simulink model "Beautiful_powertrain"  (R2024a)
settings: Solver=ode3  StartTime=0.0  StopTime=40  FixedStep=0.001  RelTol=1e-3
model workspace (MAT data in the model file):
  C_Aero_drag = 0.28
  C_rolling_resistance = 0.01
  C_rolling_resitance = 0.01
  C_viscous_damping = 0.02
  Damping_coef = 50
  Gear_ratio = 10
  J_vehicle = 2.56328
  Motor_no_load_speed = 16000
  Motor_rated_load = 150000
  Motor_rated_speed = 9000
  Motor_rotor_damping = 0.02
  Motor_rotor_inertia = 0.05
  Motor_voltage = 450
  Slope = 0
  Vehicle_Wheel_Radius = 0.358
  Vehicle_frontal_area = 2.56
  Vehicle_mass = 2000
values from neighbouring files (symbols this model uses):
  s = sprintf('    [N_diangostic_2.m]
undefined symbols (not defined in the file or in its folder): battery_builder_rtmsupport, gcbh
libraries: Batteries_lib x36, fl_lib x31, nesl_utility x24, ee_lib x3, autolibshared x2, rllib x2, sdl_lib x1
(part 1 of 6)
settings Model: Creator=bt  LastModifiedBy=konstantinosspiliotopoulos
settings SolverCC: AutoInsertRateTranBlk=on

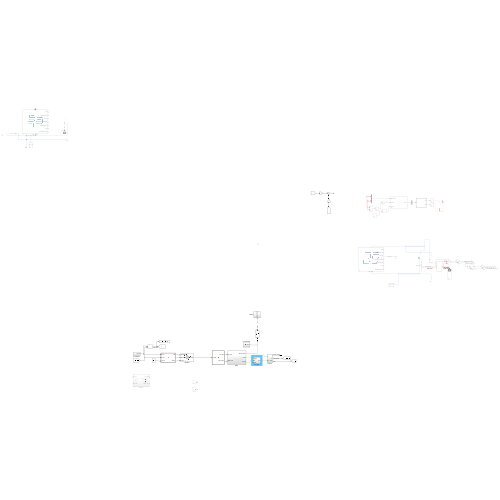
[thumbnail: Simulink's stored preview of the top-level diagram]
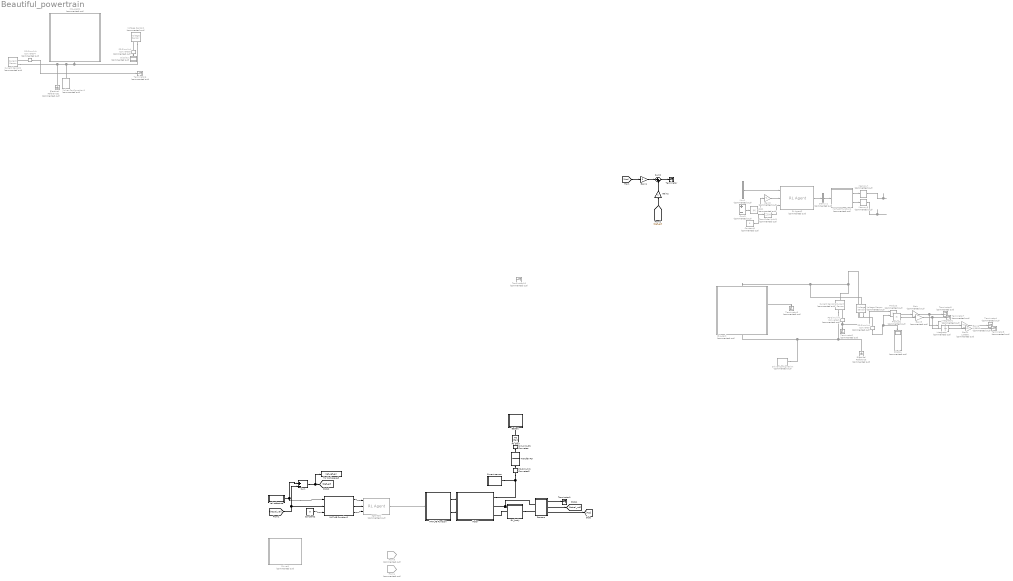
== system Beautiful_powertrain ==
  Abs1 : Abs  Commented=on  SaturateOnIntegerOverflow=off
  Battery : Subsystem
  Constant1 : Constant  Commented=on  Value=0
  Constant2 : Constant  Value=0
  Current Sensor : fl_lib/Electrical/Electrical Sensors/Current Sensor  Commented=on
  Current Sensor2 : fl_lib/Electrical/Electrical Sensors/Current Sensor  Commented=on
  Current sensor : Subsystem
  Demux1 : Demux  Commented=on  Outputs=1
  Display : Display  Commented=on
  Display1 : Display  Commented=on
  Driver1 : Subsystem  Commented=on
  EV_body : Subsystem
  Electrical Reference : fl_lib/Electrical/Electrical Elements/Electrical Reference  Commented=on
  Electrical Reference1 : fl_lib/Electrical/Electrical Elements/Electrical Reference  Commented=on
  From3 : From  Commented=on  GotoTag=Vel_ref
  From4 : From  Commented=on  GotoTag=vel_act
  Gain : Gain  Commented=on  Gain=1e-3
  Gain1 : Gain
  Gain2 : Gain
  Gain3 : Gain  Commented=on  Gain=-1
  Gain4 : Gain  Commented=on  Gain=1/3600
  Gain5 : Gain  Commented=on  Gain=1e-3
  Gain6 : Gain  Commented=on  Gain=1/3600
  ID4_pack : Subsystem  Commented=on  LoadFcn=battery_builder_rtmsupport('loadfcn',gcbh);
      settings: CopyFcn=battery_builder_rtmsupport('copyfcn',gcbh);  PreCopyFcn=battery_builder_rtmsupport('precopyfcn',gcbh);  PreDeleteFcn=battery_builder_rtmsupport('predeletefcn',gcbh);  PortSchema="{\"entries\":[{\"content\":{\"sides\":[{\"content\":{\"connectorIds\":[\"LConn1\"]},\"type\":\"ConnectorPlacement.EquallySpacedRectSide\",\"uuid\":\"ff832d46-24c2-48f3-9ca2-acbc79ffea0e\"},{\"content\":{\"connectorIds\":[\"RConn1\"],\"side\":\"RIGHT\"},\"type\":\"ConnectorPlacement.EquallySpacedRectSide\",\"uuid\":\"f1f3b13c-36d9-4e7c-bb66-ad6aba201785\"},{\"content\":{\"side\":\"TOP\"},\"type\":\"ConnectorPlacement.EquallySpacedRectSide\",\"uuid\":\"497ed55c-0d21-4aaa-b04e-04d199c99403\"},{\"content\":{\"connectorIds\":[\"Out1\",\"Out2\",\"Out3\",\"Out4\",\"Out5\",\"Out6\",\"Out7\"],\"side\":\"BOTTOM\"},\"type\":\"ConnectorPlacement.EquallySpacedRectSide\",\"uuid\":\"fb4a2477-79f0-4aed-96ce-fa2286ad26a5\"}]},\"type\":\"ConnectorPlacement.EquallySpacedConnector\",\"uuid\":\"b44e404e-c709-4efd-83da-0fbfd4cccfd0\"}],\"packageUris\":[\"http://schema.mathworks.com/mf0/Connector/R2020b\"],\"version\":\"1.0\"}"
      mask Display: image('$imagefile')
  ID4_pack1 : Subsystem  Commented=on  LoadFcn=battery_builder_rtmsupport('loadfcn',gcbh);
      settings: CopyFcn=battery_builder_rtmsupport('copyfcn',gcbh);  PreCopyFcn=battery_builder_rtmsupport('precopyfcn',gcbh);  PreDeleteFcn=battery_builder_rtmsupport('predeletefcn',gcbh);  PortSchema="{\"entries\":[{\"content\":{\"sides\":[{\"content\":{\"connectorIds\":[\"LConn1\"]},\"type\":\"ConnectorPlacement.EquallySpacedRectSide\",\"uuid\":\"ff832d46-24c2-48f3-9ca2-acbc79ffea0e\"},{\"content\":{\"connectorIds\":[\"RConn1\"],\"side\":\"RIGHT\"},\"type\":\"ConnectorPlacement.EquallySpacedRectSide\",\"uuid\":\"f1f3b13c-36d9-4e7c-bb66-ad6aba201785\"},{\"content\":{\"side\":\"TOP\"},\"type\":\"ConnectorPlacement.EquallySpacedRectSide\",\"uuid\":\"497ed55c-0d21-4aaa-b04e-04d199c99403\"},{\"content\":{\"connectorIds\":[\"Out1\",\"Out2\",\"Out3\",\"Out4\",\"Out5\",\"Out6\",\"Out7\"],\"side\":\"BOTTOM\"},\"type\":\"ConnectorPlacement.EquallySpacedRectSide\",\"uuid\":\"fb4a2477-79f0-4aed-96ce-fa2286ad26a5\"}]},\"type\":\"ConnectorPlacement.EquallySpacedConnector\",\"uuid\":\"b44e404e-c709-4efd-83da-0fbfd4cccfd0\"}],\"packageUris\":[\"http://schema.mathworks.com/mf0/Connector/R2020b\"],\"version\":\"1.0\"}"
      mask Display: image('$imagefile')
  Integrator : Integrator  Commented=on
  Integrator1 : Integrator  Commented=on
  MATLAB Function : MATLAB Function  TreatAsAtomicUnit=on
  MATLAB Function1 : MATLAB Function  Commented=on  TreatAsAtomicUnit=on
  MATLAB Function2 : MATLAB Function  TreatAsAtomicUnit=on
  Memory2 : Memory  Commented=on
  Memory3 : Memory  Commented=on
  Motor : Subsystem
  Mux1 : Mux  Commented=on  Inputs=2
  PS Gain : fl_lib/Physical Signals/Functions/PS Gain  gain=1
  PS-Simulink Converter{,1,3..4} (4 alike) : nesl_utility/PS-Simulink Converter  Commented=on  PhysicalDomain=network_engine_domain  SubClassName=ps_output  LeftPortType=input  RightPortType=output  PseudoPeriodic=off  Frequencies=[]  VectorFormat=inherit  Unit=inherit  AffineConversion=off
  PS-Simulink Converter2 : nesl_utility/PS-Simulink Converter  PhysicalDomain=network_engine_domain  SubClassName=ps_output  LeftPortType=input  RightPortType=output  PseudoPeriodic=off  Frequencies=[]  VectorFormat=inherit  Unit=inherit  AffineConversion=off
  Product : Product  Commented=on
  Product1 : Product  Commented=on
  RL Agent2 : rllib/RL Agent  Commented=on  Agent=agentObj  ExternalActionAsInput=off  ProvideLastAction=off  ProvideCumRwd=off  TreatAsDirectFeedthrough=on  UseStrictObservationDataTypes=off
  Sensors : Subsystem
  Simulink-PS Converter : nesl_utility/Simulink-PS Converter  PhysicalDomain=network_engine_domain  SubClassName=ps_input  LeftPortType=input  RightPortType=output  PseudoPeriodic=off  Frequencies=[]  NoiseDistribution=none  NoiseParameters=[]  Unit=1  AffineConversion=off  FilteringAndDerivatives=provide  SimscapeFilterOrder=1  InputFilterTimeConstant=0.001  UdotUserProvided=0
  Solver Configuration : nesl_utility/Solver Configuration  Commented=on  PhysicalDomain=network_engine_domain  SubClassName=solver  LeftPortType=input  RightPortType=generic  Tones=[]  Harmonics=[]  SimulateNoise=off  Profile=off  UseLocalSampling=off  EnableSwitchedLinearOptims=on  FrequencyDomain=off  UseCCode=off  RelTol=0.001  AbsTol=0.001  MinStep=1e-09  ToWorkspace=off  RevertToSquareIcSolve=off  NumHomotopyIterations=100  PhasorMode=off  PhasorModeNumHarmonics=1  ConsistencySolver=NEWTON_XTOL_AFTER_FTOL  IndexReductionMethod=DerivativeReplacement  DoDC=off  ResidualTolerance=1e-09  ConsistencyTolSource=GLOBAL  ConsistencyAbsTol=0.001  ConsistencyRelTol=0.001  ConsistencyTolFactor=0.001  UseLocalSolver=off  LocalSolverChoice=NE_BACKWARD_EULER_ADVANCER  ResolveIndetEquations=on  FunctionEvalNumThread=1  LocalSolverSampleTime=0.001  DoFixedCost=off  MaxNonlinIter=3  MaxModeIter=2  ComputeImpulses=off  ImpulseIterations=2  LinearAlgebra=auto  LinearAlgebraNumThread=0  EquationFormulation=NE_TIME_EF  DelaysMemoryBudget=1024  AutomaticFiltering=on  FilteringTimeConstant=0.001  PartitionStorageMethod=AS_NEEDED  PartitionMemoryBudget=1024  PartitionMethod=ROBUST  MultibodyUseLocalSolver=off  MultibodyLocalSolverChoice=ODE1  MultibodyLocalSolverSampleTime=0.001
  Solver Configuration1 : nesl_utility/Solver Configuration  Commented=on  PhysicalDomain=network_engine_domain  SubClassName=solver  LeftPortType=input  RightPortType=generic  Tones=[]  Harmonics=[]  SimulateNoise=off  Profile=off  UseLocalSampling=off  EnableSwitchedLinearOptims=on  FrequencyDomain=off  UseCCode=off  RelTol=0.001  AbsTol=0.001  MinStep=1e-09  ToWorkspace=off  RevertToSquareIcSolve=off  NumHomotopyIterations=100  PhasorMode=off  PhasorModeNumHarmonics=1  ConsistencySolver=NEWTON_XTOL_AFTER_FTOL  IndexReductionMethod=DerivativeReplacement  DoDC=off  ResidualTolerance=1e-09  ConsistencyTolSource=GLOBAL  ConsistencyAbsTol=0.001  ConsistencyRelTol=0.001  ConsistencyTolFactor=0.001  UseLocalSolver=off  LocalSolverChoice=NE_BACKWARD_EULER_ADVANCER  ResolveIndetEquations=on  FunctionEvalNumThread=1  LocalSolverSampleTime=0.001  DoFixedCost=off  MaxNonlinIter=3  MaxModeIter=2  ComputeImpulses=off  ImpulseIterations=2  LinearAlgebra=auto  LinearAlgebraNumThread=0  EquationFormulation=NE_TIME_EF  DelaysMemoryBudget=1024  AutomaticFiltering=on  FilteringTimeConstant=0.001  PartitionStorageMethod=AS_NEEDED  PartitionMemoryBudget=1024  PartitionMethod=ROBUST  MultibodyUseLocalSolver=off  MultibodyLocalSolverChoice=ODE1  MultibodyLocalSolverSampleTime=0.001
  Sum : Sum  Inputs=|+-
  Sum2 : Sum  Inputs=|++
  Sum3 : Sum  Commented=on  Inputs=+-
  Terminator : Terminator
  Terminator1 : Terminator
  Terminator{2..8,10} (8 alike) : Terminator  Commented=on
  To Workspace3 : ToWorkspace  VariableName=Veh_ref_err  SaveFormat=Structure With Time  SampleTime=-1
  Transfer Fcn : TransferFcn  Denominator=[1e-2 1]
  Vel reference : Subsystem
  Voltage Sensor : fl_lib/Electrical/Electrical Sensors/Voltage Sensor  Commented=on
  Voltage Sensor1 : fl_lib/Electrical/Electrical Sensors/Voltage Sensor  Commented=on
  Zero-Order Hold1 : ZeroOrderHold  Commented=on  SampleTime=-1
  agentObj : rllib/RL Agent  Commented=on  Agent=agentObj  ExternalActionAsInput=off  ProvideLastAction=off  ProvideCumRwd=off  TreatAsDirectFeedthrough=on  UseStrictObservationDataTypes=off
  wires:
  Sensors/3(ACC) -> [Acc]  "ACC"
  [Acc] -> Gain1/1
  Gain1/1 -> Sum2/1
  Gain2/1 -> Sum2/2
  Sum2/1 -> Terminator/1
  Vel reference/1(Vel_ref) -> MATLAB Function2/1(Vel_ref), Sum/1
  [Actual_vel] -> Sum/2, MATLAB Function2/2(Vel_act)
  Memory3/1 -> ?
  MATLAB Function1/2(brk) -> Memory3/1
  Memory2/1 -> ?
  MATLAB Function1/1(acc) -> Memory2/1
  Demux1/1 -> MATLAB Function1/1(u)
  RL Agent2/1 -> Demux1/1
  Zero-Order Hold1/1 -> RL Agent2/3
  Constant1/1 -> Zero-Order Hold1/1
  Gain3/1 -> RL Agent2/2
  Abs1/1 -> Gain3/1
  Sum3/1 -> Abs1/1
  Mux1/1 -> RL Agent2/1
  ? -> Sum3/2
  ? -> Mux1/2
  ? -> Sum3/1
  ? -> Mux1/1
  Sensors/1(I) -> Terminator1/1  "Motor_omega"
  Sensors/2(O) -> [Actual_vel]  "ACTUAL VEL"
  Sum/1 -> To Workspace3/1, [Ref_err]  "REF_ERR"
  [Ref_err] -> Gain2/1
  PS-Simulink Converter/1 -> Product/2, Display/1  "Bat_Voltage"
  PS-Simulink Converter1/1 -> Terminator2/1, Product/1  "Bat_current"
  Product/1 -> Gain/1
  Gain/1 -> Integrator/1, Terminator3/1  "Bat_power [kW]"
  Integrator/1 -> Gain4/1
  Gain4/1 -> Terminator4/1  "Energy used [kWh]"
  PS-Simulink Converter2/1 -> Transfer Fcn/1
  Transfer Fcn/1 -> Simulink-PS Converter/1
  ID4_pack/3(socCell) -> Terminator5/1  "Bat_soc"
  PS-Simulink Converter3/1 -> Display1/1  "Bat_V"
  PS-Simulink Converter4/1 -> Terminator6/1  "Bat_I"
  ? -> Product1/2  "Bat_Voltage"
  Gain5/1 -> Integrator1/1, Terminator7/1  "Bat_power [kW]"
  ? -> ?  "Bat_Voltage"
  Product1/1 -> Gain5/1
  ? -> Product1/1  "Bat_current"
  Gain6/1 -> Terminator8/1  "Energy used [kWh]"
  Integrator1/1 -> Gain6/1
  MATLAB Function/1(Acc_cmd) -> Motor/1(Acc_cmd)
  MATLAB Function/2(Brake_cmd) -> Motor/2(Brake_cmd)
  Constant2/1 -> MATLAB Function2/3(u_used)
  MATLAB Function2/1(obs) -> agentObj/1
  MATLAB Function2/2(r) -> agentObj/2
  MATLAB Function2/3(isdone) -> agentObj/3
  agentObj/1 -> MATLAB Function/1(u_scalar)
  connections:
  Motor/RConn1 -- Current sensor/LConn1 -- PS-Simulink Converter2/LConn1
  EV_body/LConn1 -- Sensors/LConn1 -- Motor/RConn2
  EV_body/LConn2 -- Motor/RConn3
  EV_body/RConn1 -- Sensors/LConn2
  Electrical Reference/LConn1 -- Current Sensor/RConn2 -- Solver Configuration/RConn1 -- ID4_pack/RConn1
  PS-Simulink Converter/LConn1 -- Voltage Sensor/RConn1
  Voltage Sensor/LConn1 -- ID4_pack/LConn1 -- Current Sensor/LConn1 -- Voltage Sensor/RConn2
  PS-Simulink Converter1/LConn1 -- Current Sensor/RConn1
  Simulink-PS Converter/RConn1 -- PS Gain/LConn1
  Electrical Reference1/LConn1 -- Current Sensor2/RConn2 -- Voltage Sensor1/RConn2 -- ID4_pack1/RConn1 -- Solver Configuration1/RConn1
  PS-Simulink Converter3/LConn1 -- Voltage Sensor1/RConn1
  PS-Simulink Converter4/LConn1 -- Current Sensor2/RConn1
  PS Gain/RConn1 -- Battery/RConn1

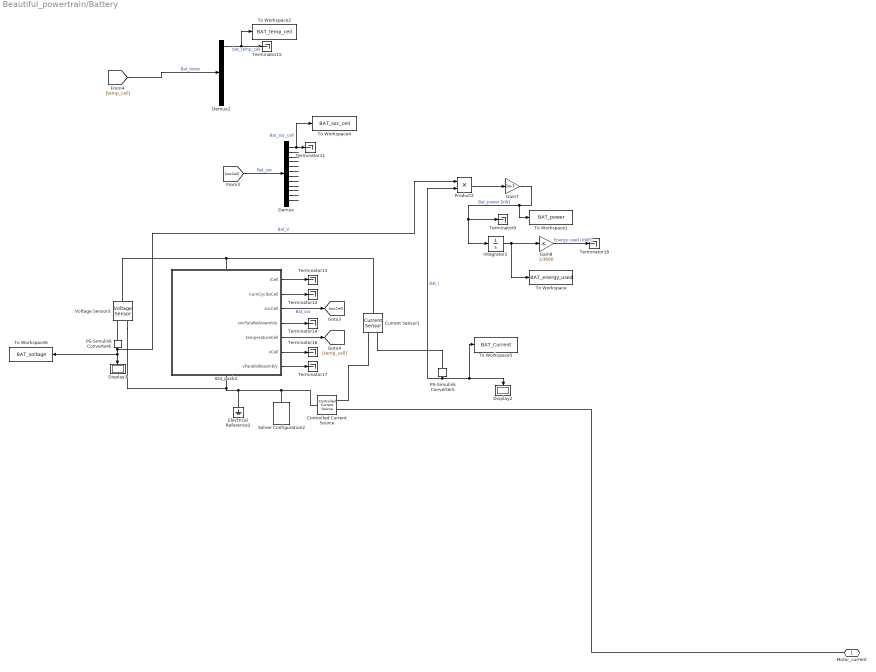
== system Beautiful_powertrain/Battery ==
  Controlled Current Source : fl_lib/Electrical/Electrical Sources/Controlled Current Source
  Current Sensor1 : fl_lib/Electrical/Electrical Sensors/Current Sensor
  Demux : Demux  Outputs=12
  Demux2 : Demux  Outputs=12
  Display2 : Display
  Display3 : Display
  Electrical Reference2 : fl_lib/Electrical/Electrical Elements/Electrical Reference
  Gain7 : Gain  Gain=1e-3
  Gain8 : Gain  Gain=1/3600
  ID4_pack2 : Subsystem  LoadFcn=battery_builder_rtmsupport('loadfcn',gcbh);
      settings: CopyFcn=battery_builder_rtmsupport('copyfcn',gcbh);  PreCopyFcn=battery_builder_rtmsupport('precopyfcn',gcbh);  PreDeleteFcn=battery_builder_rtmsupport('predeletefcn',gcbh);  PortSchema="{\"entries\":[{\"content\":{\"sides\":[{\"content\":{\"connectorIds\":[\"LConn1\"]},\"type\":\"ConnectorPlacement.EquallySpacedRectSide\",\"uuid\":\"ff832d46-24c2-48f3-9ca2-acbc79ffea0e\"},{\"content\":{\"connectorIds\":[\"RConn1\"],\"side\":\"RIGHT\"},\"type\":\"ConnectorPlacement.EquallySpacedRectSide\",\"uuid\":\"f1f3b13c-36d9-4e7c-bb66-ad6aba201785\"},{\"content\":{\"side\":\"TOP\"},\"type\":\"ConnectorPlacement.EquallySpacedRectSide\",\"uuid\":\"497ed55c-0d21-4aaa-b04e-04d199c99403\"},{\"content\":{\"connectorIds\":[\"Out1\",\"Out2\",\"Out3\",\"Out4\",\"Out5\",\"Out6\",\"Out7\"],\"side\":\"BOTTOM\"},\"type\":\"ConnectorPlacement.EquallySpacedRectSide\",\"uuid\":\"fb4a2477-79f0-4aed-96ce-fa2286ad26a5\"}]},\"type\":\"ConnectorPlacement.EquallySpacedConnector\",\"uuid\":\"b44e404e-c709-4efd-83da-0fbfd4cccfd0\"}],\"packageUris\":[\"http://schema.mathworks.com/mf0/Connector/R2020b\"],\"version\":\"1.0\"}"
      mask Display: image('$imagefile')
  Integrator2 : Integrator
  PS-Simulink Converter5 : nesl_utility/PS-Simulink Converter  PhysicalDomain=network_engine_domain  SubClassName=ps_output  LeftPortType=input  RightPortType=output  PseudoPeriodic=off  Frequencies=[]  VectorFormat=inherit  Unit=inherit  AffineConversion=off
  PS-Simulink Converter6 : nesl_utility/PS-Simulink Converter  PhysicalDomain=network_engine_domain  SubClassName=ps_output  LeftPortType=input  RightPortType=output  PseudoPeriodic=off  Frequencies=[]  VectorFormat=inherit  Unit=inherit  AffineConversion=off
  Product2 : Product
  Solver Configuration2 : nesl_utility/Solver Configuration  PhysicalDomain=network_engine_domain  SubClassName=solver  LeftPortType=input  RightPortType=generic  Tones=[]  Harmonics=[]  SimulateNoise=off  Profile=off  UseLocalSampling=off  EnableSwitchedLinearOptims=on  FrequencyDomain=off  UseCCode=off  RelTol=0.001  AbsTol=0.001  MinStep=1e-09  ToWorkspace=off  RevertToSquareIcSolve=off  NumHomotopyIterations=100  PhasorMode=off  PhasorModeNumHarmonics=1  ConsistencySolver=NEWTON_XTOL_AFTER_FTOL  IndexReductionMethod=DerivativeReplacement  DoDC=off  ResidualTolerance=1e-09  ConsistencyTolSource=GLOBAL  ConsistencyAbsTol=0.001  ConsistencyRelTol=0.001  ConsistencyTolFactor=0.001  UseLocalSolver=off  LocalSolverChoice=NE_BACKWARD_EULER_ADVANCER  ResolveIndetEquations=on  FunctionEvalNumThread=1  LocalSolverSampleTime=0.001  DoFixedCost=off  MaxNonlinIter=3  MaxModeIter=2  ComputeImpulses=off  ImpulseIterations=2  LinearAlgebra=auto  LinearAlgebraNumThread=0  EquationFormulation=NE_TIME_EF  DelaysMemoryBudget=1024  AutomaticFiltering=on  FilteringTimeConstant=0.001  PartitionStorageMethod=AS_NEEDED  PartitionMemoryBudget=1024  PartitionMethod=ROBUST  MultibodyUseLocalSolver=off  MultibodyLocalSolverChoice=ODE1  MultibodyLocalSolverSampleTime=0.001
  Terminator{9,11..18} (9 alike) : Terminator
  To Workspace : ToWorkspace  VariableName=BAT_energy_used  SaveFormat=Structure With Time  SampleTime=-1
  To Workspace1 : ToWorkspace  VariableName=BAT_power  SaveFormat=Structure With Time  SampleTime=-1
  To Workspace2 : ToWorkspace  VariableName=BAT_temp_cell  SaveFormat=Structure With Time  SampleTime=-1
  To Workspace4 : ToWorkspace  VariableName=BAT_soc_cell  SaveFormat=Structure With Time  SampleTime=-1
  To Workspace5 : ToWorkspace  VariableName=BAT_Current  SaveFormat=Structure With Time  SampleTime=-1
  To Workspace6 : ToWorkspace  VariableName=BAT_voltage  SaveFormat=Structure With Time  SampleTime=-1
  Voltage Sensor3 : fl_lib/Electrical/Electrical Sensors/Voltage Sensor
  Motor_current : PMIOPort  Side=Right
  wires:
  Demux/7 -> ?
  Demux/5 -> ?
  Demux/4 -> ?
  Demux/8 -> ?
  Demux/10 -> ?
  [socCell] -> Demux/1  "Bat_soc"
  ID4_pack2/3(socCell) -> [socCell]  "Bat_soc"
  [temp_cell] -> Demux2/1  "Bat_temp"
  ID4_pack2/2(numCyclesCell) -> Terminator12/1
  Demux/11 -> ?
  Demux/6 -> ?
  ID4_pack2/6(vCell) -> Terminator16/1
  Demux/2 -> ?
  Demux2/1 -> Terminator15/1, To Workspace2/1  "bat_temp_cell"
  ID4_pack2/4(socParallelAssembly) -> Terminator14/1
  ID4_pack2/1(iCell) -> Terminator13/1
  Demux/1 -> To Workspace4/1, Terminator11/1  "Bat_soc_cell"
  Gain8/1 -> Terminator18/1  "Energy used [kWh]"
  Product2/1 -> Gain7/1
  PS-Simulink Converter6/1 -> To Workspace6/1, Display3/1, Product2/1  "Bat_V"
  Demux/12 -> ?
  Demux/3 -> ?
  ID4_pack2/5(temperatureCell) -> [temp_cell]
  Integrator2/1 -> Gain8/1, To Workspace/1
  ID4_pack2/7(vParallelAssembly) -> Terminator17/1
  Demux/9 -> ?
  Gain7/1 -> To Workspace1/1, Integrator2/1, Terminator9/1  "Bat_power [kW]"
  PS-Simulink Converter5/1 -> Product2/2, To Workspace5/1, Display2/1  "Bat_I"
  connections:
  Current Sensor1/RConn1 -- PS-Simulink Converter5/LConn1
  Current Sensor1/RConn2 -- Controlled Current Source/RConn2
  PS-Simulink Converter6/LConn1 -- Voltage Sensor3/RConn1
  Voltage Sensor3/LConn1 -- Current Sensor1/LConn1 -- ID4_pack2/LConn1
  Motor_current/RConn1 -- Controlled Current Source/RConn1
  ID4_pack2/RConn1 -- Voltage Sensor3/RConn2 -- Controlled Current Source/LConn1 -- Solver Configuration2/RConn1 -- Electrical Reference2/LConn1

== system Beautiful_powertrain/Current sensor ==
  PS Gain : fl_lib/Physical Signals/Functions/PS Gain  gain=-1
  PS-Simulink Converter2 : nesl_utility/PS-Simulink Converter  PhysicalDomain=network_engine_domain  SubClassName=ps_output  LeftPortType=input  RightPortType=output  PseudoPeriodic=off  Frequencies=[]  VectorFormat=inherit  Unit=inherit  AffineConversion=off
  Terminator3 : Terminator
  To Workspace6 : ToWorkspace  VariableName=Btry_I_in  SaveFormat=Structure With Time  SampleTime=-1
  I_motor : PMIOPort  Side=Left
  wires:
  PS-Simulink Converter2/1 -> To Workspace6/1, Terminator3/1  "Btry_I_in"
  connections:
  PS Gain/LConn1 -- I_motor/RConn1
  PS-Simulink Converter2/LConn1 -- PS Gain/RConn1

== system Beautiful_powertrain/Driver1 ==
  Vel_ref : Inport
  Vel_fdbk : Inport  Port=2
  Constant2 : Constant  Value=0
  Longitudinal Driver : autolibshared/Longitudinal Driver  extAccelOvr=off  extDecelOvr=off  extAccelHld=off  extDecelHld=off  extAccelZero=off  extDecelZero=off  cntrlType=PI  shftType=None  velUnits=m/s  gearOut=off  Kp=15  Ki=1  Kff=.05  Kg=.01  VehVelVec=[0 100]  KffVec=[.1 .1]  KpVec=[10 10]  KiVec=[5 5]  KgVec=[0 0]  m=1500  Kpt=3000  tau=.1  L=2  aR=200  bR=2.5  cR=.5  g=9.81  vnom=100  Kaw=.1  tauerr=.03  tauPt=2  GearInit=0  tShift=.1  pdlVec=[0.1 0.4 0.5 0.9]  upShftTbl=[-1 12.9375 26.4375 39.9375 51.18749999999999 62.4375 72.84375 83.25;-1 16.3125 29.8125 43.3125 54.5624 65.8125 76.78125 87.75;-1 19.6875 33.1875 46.68749999999999 57.9375 69.1875 80.71875 92.25;-1 33 52.5 77.25 100.5 138.75 161.875 185]  dwnShftTbl=[1 9.5625 23.0625 36.5625 47.8125 59.0625 68.90625 78.75;1 12.9375 26.4375 39.9375 51.18749999999999 62.4375 72.84375 83.25;1 16.3125 29.8125 43.3125 54.562499 65.8125 76.78125 87.75;1 19.6875 33.1875 46.68749999999999 57.9375 69.1875 80.71875 92.25]  tClutch=.5  tRev=.5  tPark=120  aMode=1  UpGearVec="[0  1  2  3  4  5  6  7]"  DownGearVec="[1  2  3  4  5  6  7  8]"
  To Workspace1 : ToWorkspace  VariableName=Driver_acc_cmd  SaveFormat=Structure With Time  SampleTime=-1
  To Workspace2 : ToWorkspace  VariableName=Driver_brake_cmd1  SaveFormat=Structure With Time  SampleTime=-1
  Acc_cmd : Outport
  Brake_cmd : Outport  Port=2
  wires:
  Longitudinal Driver/2 -> Acc_cmd/1, To Workspace1/1  "Acc_cmd"
  Longitudinal Driver/3 -> To Workspace2/1, Brake_cmd/1  "Brake_cmd"
  Constant2/1 -> Longitudinal Driver/3
  Longitudinal Driver/1 -> ?
  Vel_ref/1 -> Longitudinal Driver/1
  Vel_fdbk/1 -> Longitudinal Driver/2

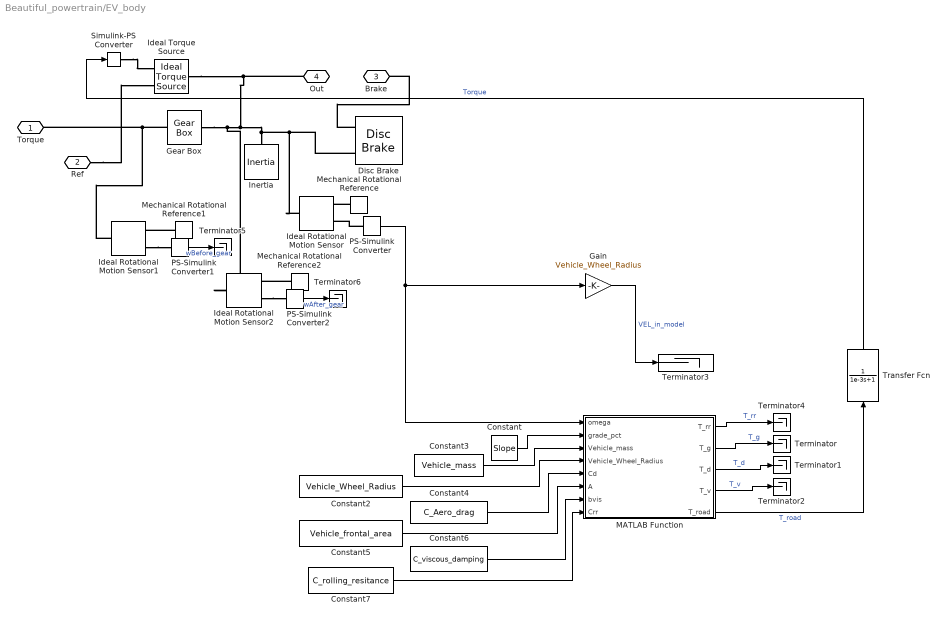
== system Beautiful_powertrain/EV_body ==
  Constant : Constant  Value=Slope
  Constant2 : Constant  Value=Vehicle_Wheel_Radius
  Constant3 : Constant  Value=Vehicle_mass
  Constant4 : Constant  Value=C_Aero_drag
  Constant5 : Constant  Value=Vehicle_frontal_area
  Constant6 : Constant  Value=C_viscous_damping
  Constant7 : Constant  Value=C_rolling_resitance
  Disc Brake : sdl_lib/Brakes & Detents/Rotational/Disc Brake  r_mean=150 mm  bore=10 mm  n_pads=2  enable_faults=simscape.enum.onoff.off  faulted_pressure=0 bar  thermal_port=simscape.enum.thermaleffects.omit  mu_static=0.9  mu_coulomb=0.7  temperature_TLU=[280, 300, 320] K  mu_static_TLU=[.9, .8, .7]  mu_coulomb_TLU=[.8, .7, .6]  brkwy_vel=0.1 rad/s  visc_coef=0 N*m*s/rad  thermal_mass=50 kJ/K  temperature_specify=off  temperature_priority=High  temperature=300 K  temperature_nominal_specify=off  temperature_nominal_value=1  temperature_nominal_unit=K
  Gain : Gain  Gain=Vehicle_Wheel_Radius
  Gear Box : fl_lib/Mechanical/Mechanisms/Gear Box  ratio=Gear_ratio  t_in_specify=off  t_in_priority=None  t_in=0 N*m  t_in_nominal_specify=off  t_in_nominal_value=1  t_in_nominal_unit=N*m  t_out_specify=off  t_out_priority=None  t_out=0 N*m  t_out_nominal_specify=off  t_out_nominal_value=1  t_out_nominal_unit=N*m
  Ideal Rotational Motion Sensor : fl_lib/Mechanical/Mechanical Sensors/Ideal Rotational Motion Sensor  reference=foundation.enum.MeasurementReference.difference  acceleration_port=false  velocity_port=true  position_port=false  wrap_angle=false  offset=0 rad
      settings: InternalSimscapePortConfiguration="{\"Bottom\":[],\"Left\":[{\"id\":\"R\",\"label\":\"R\",\"type\":\"foundation.mechanical.rotational.rotational\"}],\"Right\":[{\"id\":\"C\",\"label\":\"C\",\"type\":\"foundation.mechanical.rotational.rotational\"},{\"id\":\"W\",\"label\":\"W\",\"type\":\"output\"}],\"Top\":[]}"
  Ideal Rotational Motion Sensor1 : fl_lib/Mechanical/Mechanical Sensors/Ideal Rotational Motion Sensor  reference=foundation.enum.MeasurementReference.difference  acceleration_port=false  velocity_port=true  position_port=false  wrap_angle=false  offset=0 rad
      settings: InternalSimscapePortConfiguration="{\"Bottom\":[],\"Left\":[{\"id\":\"R\",\"label\":\"R\",\"type\":\"foundation.mechanical.rotational.rotational\"}],\"Right\":[{\"id\":\"C\",\"label\":\"C\",\"type\":\"foundation.mechanical.rotational.rotational\"},{\"id\":\"W\",\"label\":\"W\",\"type\":\"output\"}],\"Top\":[]}"
  Ideal Rotational Motion Sensor2 : fl_lib/Mechanical/Mechanical Sensors/Ideal Rotational Motion Sensor  reference=foundation.enum.MeasurementReference.difference  acceleration_port=false  velocity_port=true  position_port=false  wrap_angle=false  offset=0 rad
      settings: InternalSimscapePortConfiguration="{\"Bottom\":[],\"Left\":[{\"id\":\"R\",\"label\":\"R\",\"type\":\"foundation.mechanical.rotational.rotational\"}],\"Right\":[{\"id\":\"C\",\"label\":\"C\",\"type\":\"foundation.mechanical.rotational.rotational\"},{\"id\":\"W\",\"label\":\"W\",\"type\":\"output\"}],\"Top\":[]}"
  Ideal Torque Source : fl_lib/Mechanical/Mechanical Sources/Ideal Torque Source
  Inertia : fl_lib/Mechanical/Rotational Elements/Inertia  inertia=J_vehicle kg*m^2  num_ports=foundation.enum.numPorts2.one  w_specify=off  w_priority=High  w=0 rad/s  w_nominal_specify=off  w_nominal_value=1  w_nominal_unit=rad/s  t_specify=off  t_priority=None  t=0 N*m  t_nominal_specify=off  t_nominal_value=1  t_nominal_unit=N*m
  MATLAB Function : MATLAB Function  TreatAsAtomicUnit=on
  Mechanical Rotational Reference : fl_lib/Mechanical/Rotational Elements/Mechanical Rotational Reference
  Mechanical Rotational Reference1 : fl_lib/Mechanical/Rotational Elements/Mechanical Rotational Reference
  Mechanical Rotational Reference2 : fl_lib/Mechanical/Rotational Elements/Mechanical Rotational Reference
  PS-Simulink Converter : nesl_utility/PS-Simulink Converter  PhysicalDomain=network_engine_domain  SubClassName=ps_output  LeftPortType=input  RightPortType=output  PseudoPeriodic=off  Frequencies=[]  VectorFormat=inherit  Unit=inherit  AffineConversion=off
  PS-Simulink Converter1 : nesl_utility/PS-Simulink Converter  PhysicalDomain=network_engine_domain  SubClassName=ps_output  LeftPortType=input  RightPortType=output  PseudoPeriodic=off  Frequencies=[]  VectorFormat=inherit  Unit=inherit  AffineConversion=off
  PS-Simulink Converter2 : nesl_utility/PS-Simulink Converter  PhysicalDomain=network_engine_domain  SubClassName=ps_output  LeftPortType=input  RightPortType=output  PseudoPeriodic=off  Frequencies=[]  VectorFormat=inherit  Unit=inherit  AffineConversion=off
  Simulink-PS Converter : nesl_utility/Simulink-PS Converter  PhysicalDomain=network_engine_domain  SubClassName=ps_input  LeftPortType=input  RightPortType=output  PseudoPeriodic=off  Frequencies=[]  NoiseDistribution=none  NoiseParameters=[]  Unit=1  AffineConversion=off  FilteringAndDerivatives=provide  SimscapeFilterOrder=1  InputFilterTimeConstant=0.001  UdotUserProvided=0
  Terminator{,1..6} (7 alike) : Terminator
  Transfer Fcn : TransferFcn  Denominator=[1e-3 1]
  Torque : PMIOPort  Side=Left
  Ref : PMIOPort  Port=2  Side=Left
  Brake : PMIOPort  Port=3  Side=Left
  Out : PMIOPort  Port=4  Side=Right
  wires:
  Constant/1 -> MATLAB Function/2(grade_pct)
  Constant3/1 -> MATLAB Function/3(Vehicle_mass)
  MATLAB Function/2(T_g) -> Terminator/1  "T_g"
  MATLAB Function/3(T_d) -> Terminator1/1  "T_d"
  MATLAB Function/4(T_v) -> Terminator2/1  "T_v"
  MATLAB Function/5(T_road) -> Transfer Fcn/1  "T_road"
  MATLAB Function/1(T_rr) -> Terminator4/1  "T_rr"
  Constant4/1 -> MATLAB Function/5(Cd)
  Constant2/1 -> MATLAB Function/4(Vehicle_Wheel_Radius)
  Constant5/1 -> MATLAB Function/6(A)
  Constant6/1 -> MATLAB Function/7(bvis)
  Constant7/1 -> MATLAB Function/8(Crr)
  Gain/1 -> Terminator3/1  "VEL_in_model"
  Transfer Fcn/1 -> Simulink-PS Converter/1  "Torque"
  PS-Simulink Converter1/1 -> Terminator5/1  "wBefore_gear"
  PS-Simulink Converter2/1 -> Terminator6/1  "wAfter_gear"
  PS-Simulink Converter/1 -> MATLAB Function/1(omega), Gain/1
  connections:
  Gear Box/LConn1 -- Ideal Rotational Motion Sensor1/LConn1 -- Torque/RConn1
  Gear Box/RConn1 -- Ideal Rotational Motion Sensor2/LConn1 -- Out/RConn1 -- Ideal Torque Source/LConn1 -- Ideal Rotational Motion Sensor/LConn1 -- Disc Brake/LConn2 -- Inertia/LConn1
  Disc Brake/LConn1 -- Brake/RConn1
  Simulink-PS Converter/RConn1 -- Ideal Torque Source/RConn1
  PS-Simulink Converter/LConn1 -- Ideal Rotational Motion Sensor/RConn2
  Ref/RConn1 -- Ideal Torque Source/RConn2
  Mechanical Rotational Reference/LConn1 -- Ideal Rotational Motion Sensor/RConn1
  Mechanical Rotational Reference1/LConn1 -- Ideal Rotational Motion Sensor1/RConn1
  Ideal Rotational Motion Sensor1/RConn2 -- PS-Simulink Converter1/LConn1
  Mechanical Rotational Reference2/LConn1 -- Ideal Rotational Motion Sensor2/RConn1
  Ideal Rotational Motion Sensor2/RConn2 -- PS-Simulink Converter2/LConn1
